simulink model "test2"  (R2024b)
settings: Solver=ode4  StartTime=0.0  StopTime=10.0  FixedStep=0.001  MaxStep=1e-3  RelTol=1e-3
settings Model: Creator=Hoan  LastModifiedBy=Hoan

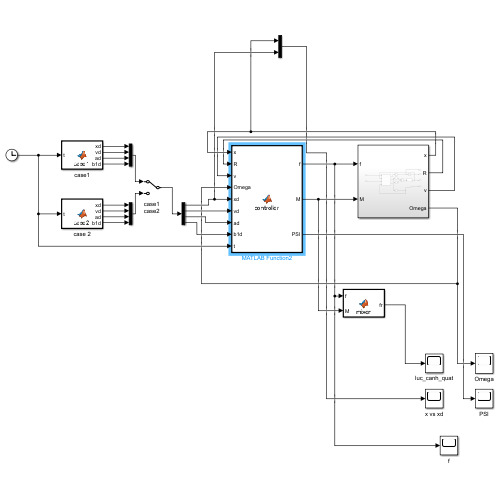
[thumbnail: Simulink's stored preview of the top-level diagram]
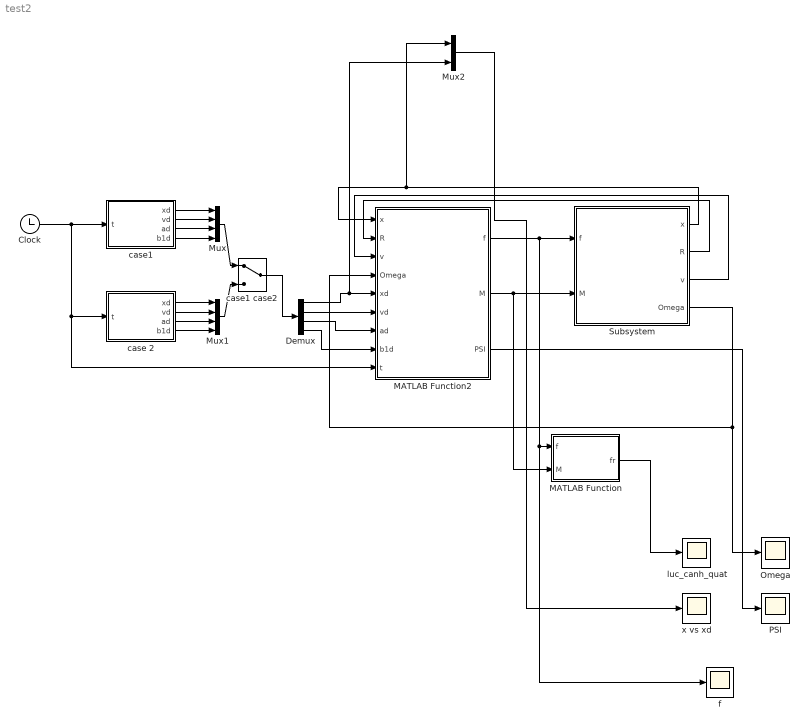
== system test2 ==
  Clock : Clock
  Demux : Demux
  MATLAB Function : MATLAB Function  TreatAsAtomicUnit=on
  MATLAB Function2 : MATLAB Function  TreatAsAtomicUnit=on
  Mux : Mux
  Mux1 : Mux
  Mux2 : Mux  Inputs=2
  Omega : Scope
  PSI : Scope
  Subsystem : Subsystem
  case 2 : MATLAB Function  TreatAsAtomicUnit=on
  case1 : MATLAB Function  TreatAsAtomicUnit=on
  "case1 case2 " : ManualSwitch
  f : Scope
  luc_canh_quat : Scope
  x vs xd : Scope
  wires:
  case1/1(xd) -> Mux/1
  case1/2(vd) -> Mux/2
  case1/3(ad) -> Mux/3
  case1/4(b1d) -> Mux/4
  case 2/1(xd) -> Mux1/1
  case 2/2(vd) -> Mux1/2
  case 2/3(ad) -> Mux1/3
  case 2/4(b1d) -> Mux1/4
  Mux/1 -> "case1 case2 "/1
  Mux1/1 -> "case1 case2 "/2
  "case1 case2 "/1 -> Demux/1
  Demux/1 -> MATLAB Function2/5(xd), Mux2/2
  Demux/3 -> MATLAB Function2/7(ad)
  Demux/2 -> MATLAB Function2/6(vd)
  Demux/4 -> MATLAB Function2/8(b1d)
  Clock/1 -> MATLAB Function2/9(t), case 2/1(t), case1/1(t)
  MATLAB Function2/1(f) -> f/1, MATLAB Function/1(f), Subsystem/1(f)
  MATLAB Function2/2(M) -> MATLAB Function/2(M), Subsystem/2(M)
  Subsystem/1(x) -> Mux2/1, MATLAB Function2/1(x)
  Subsystem/2(R) -> MATLAB Function2/2(R)
  Subsystem/4(Omega) -> MATLAB Function2/4(Omega), Omega/1
  Subsystem/3(v) -> MATLAB Function2/3(v)
  MATLAB Function/1(fr) -> luc_canh_quat/1
  MATLAB Function2/3(PSI) -> PSI/1
  Mux2/1 -> x vs xd/1

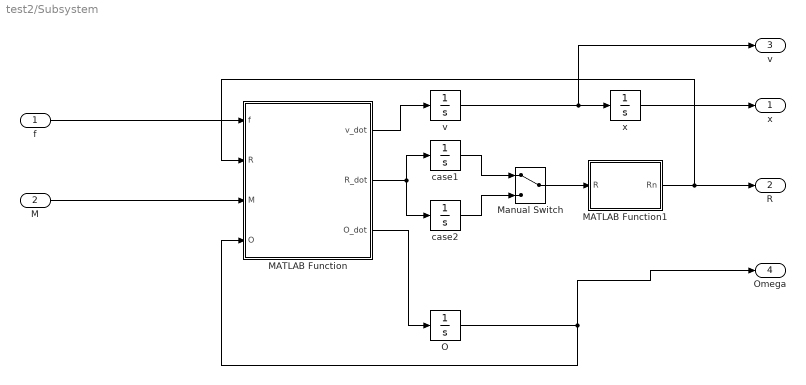
== system test2/Subsystem ==
  f : Inport
  M : Inport  Port=2
  " O" : Integrator  InitialCondition=[0;0;0]
  " v " : Integrator  InitialCondition=[0;0;0]
  " x" : Integrator  InitialCondition=[0;0;0]
  MATLAB Function : MATLAB Function  TreatAsAtomicUnit=on
  MATLAB Function1 : MATLAB Function  TreatAsAtomicUnit=on
  Manual Switch : ManualSwitch
  case1 : Integrator  InitialCondition=eye(3)
  "case2 " : Integrator  InitialCondition=[1 0 0 ; 0 -0.9995 -0.0314 ; 0 0.0314 -0.9995 ]
  x : Outport
  R : Outport  Port=2
  v : Outport  Port=3
  Omega : Outport  Port=4
  wires:
  MATLAB Function/3(O_dot) -> " O"/1
  MATLAB Function/2(R_dot) -> case1/1, "case2 "/1
  MATLAB Function/1(v_dot) -> " v "/1
  MATLAB Function1/1(Rn) -> MATLAB Function/2(R), R/1
  M/1 -> MATLAB Function/3(M)
  f/1 -> MATLAB Function/1(f)
  case1/1 -> Manual Switch/1
  "case2 "/1 -> Manual Switch/2
  Manual Switch/1 -> MATLAB Function1/1(R)
  " O"/1 -> Omega/1, MATLAB Function/4(O)
  " v "/1 -> v/1, " x"/1
  " x"/1 -> x/1

== matlab function test2/case 2 ==
  data: t input; xd output; vd output; ad output; b1d output
function [xd,vd,ad,b1d] = case2(t) %#ok<INUSD>
% Hover (Case 2)
xd  = [0;0;0];
vd  = [0;0;0];
ad  = [0;0;0];
b1d = [1;0;0];
end

== matlab function test2/case1 ==
  data: t input; xd output; vd output; ad output; b1d output
function [xd,vd,ad,b1d] = case1(t)
% Desired trajectory (Case 1)
xd = [0.4*t;0.4*sin(pi*t);-0.6*cos(pi*t)];

vd = [0.4;0.4*pi*cos(pi*t);0.6*pi*sin(pi*t)];

ad = [0;-0.4*pi*pi*sin(pi*t); 0.6*pi*pi*cos(pi*t)];

b1d = [cos(pi*t); sin(pi*t); 0];
end

== matlab function test2/MATLAB Function2 ==
  settings: updateMethod=DISCRETE
  data: x input; f output; R input; v input; Omega input; xd input; vd input; ad input; b1d input; M output; PSI output; t input
function [f, M, PSI] = controller(x, R, v, Omega, xd, vd, ad, b1d, t)
% Outputs:
%   f   : total thrust (N)
%   M   : body moment (N*m), 3x1
%   PSI : attitude configuration error function

% -------- parameters --------
m = 4.34;
g = 9.81;
J = diag([0.0820 0.0845 0.1377]);

% Gains (force-based): scale with m to keep similar closed-loop behavior
k_x = 16*m;
k_v = 5.6*m;
k_R = 8.81;
k_O = 2.54;

e3 = [0;0;1];

% -------- reshape safety --------
x     = x(:);   v     = v(:);
xd    = xd(:);  vd    = vd(:);  ad = ad(:);
Omega = Omega(:);
b1d   = b1d(:);

% -------- translational control --------
e_x = x - xd;
e_v = v - vd;

H = -k_x*e_x - k_v*e_v - m*g*e3 + m*ad;     


persistent b2d_prev
if isempty(b2d_prev)
    b2d_prev = [0;1;0];
end

% b3d
nH = norm(H);
if nH < 1e-9
    b3d = e3;
else
    b3d = -H / nH;
end

% normalize b1d
nb1 = norm(b1d);
if nb1 < 1e-9
    b1d = [1;0;0];
else
    b1d = b1d / nb1;
end

% smooth construction of b2d
Z = cross(b3d, b1d);

if norm(Z) < 1e-6
    % đừng đổi tmp đột ngột nữa, giữ hướng trước đó
    b2d = b2d_prev;
else
    b2d = Z / norm(Z);

    % giữ liên tục dấu của b2d, tránh flip 180 độ
    if dot(b2d, b2d_prev) < 0
        b2d = -b2d;
    end
end

% rebuild orthonormal basis
b1c = cross(b2d, b3d);
b1c = b1c / norm(b1c);

b2d = cross(b3d, b1c);
b2d = b2d / norm(b2d);

R_d = [b1c, b2d, b3d];

% lưu lại cho bước sau
b2d_prev = b2d;


% ensure det(Rd)=+1
[U,~,V] = svd(R_d);
R_d = U*V';
if det(R_d) < 0
    U(:,3) = -U(:,3);
    R_d = U*V';
end%

% ---------- desired angular velocity Omega_d, Omega_dot_d ----------
persistent t_prev Rd_prev Omegad_prev
if isempty(t_prev)
    t_prev = t;
    Rd_prev = R_d;
    Omegad_prev = [0;0;0];
    Omega_d = [0;0;0];
    Omega_dot_d = [0;0;0];
else
    dt = t - t_prev;
    if dt <= 1e-6
        Omega_d = Omegad_prev;
        Omega_dot_d = [0;0;0];
    else
        Rdot_d = (R_d - Rd_prev)/dt;
        W = R_d' * Rdot_d;
        W = 0.5*(W - W');      % skew
        Omega_d = vee(W);
        Omega_dot_d = (Omega_d - Omegad_prev)/dt;

        t_prev = t;
        Rd_prev = R_d;
        Omegad_prev = Omega_d;
    end
end
% -------- attitude errors --------
e_R = 0.5 * vee(R_d'*R - R'*R_d);
e_O = Omega - R'*R_d*Omega_d;

% -------- thrust and moment --------
f = -H'*(R*e3);

gyro = cross(Omega, J*Omega);
M = -k_R*e_R - k_O*e_O + gyro...
    - J*( hat(Omega)*R'*R_d*Omega_d - R'*R_d*Omega_dot_d );

% -------- PSI --------
PSI = 0.5 * trace(eye(3) - R_d'*R);

end

% ===== helpers =====
function S = hat(w)
w = w(:);
S = [   0   -w(3)  w(2);
      w(3)    0   -w(1);
     -w(2)  w(1)    0  ];
end

function w = vee(S)
w = [S(3,2); S(1,3); S(2,1)];
end

== matlab function test2/MATLAB Function ==
  data: f input; fr output; M input
function fr = mixer(f, M)
% Map total thrust & moments to rotor thrusts
% [f; Mx; My; Mz] = A * [f1; f2; f3; f4]
d = 0.315;
c = 8.004e-4;   % tau/thrust ratio (m)

A = [ 1  1  1  1;
      0 -d  0  d;
      d  0 -d  0;
      -c c -c c];

fr = A \ [f; M(:)];
end

== matlab function test2/Subsystem/MATLAB Function ==
  data: f input; v_dot output; R input; M input; O input; R_dot output; O_dot output
function [v_dot, R_dot, O_dot] = QuadDy(f, R, M, O)
% Quadrotor rigid-body dynamics (body rates)
m = 4.34;
g = 9.81;
J = diag([0.0820 0.0845 0.1377]);
e3 = [0;0;1];

O = O(:);
M = M(:);

% translation
v_dot = (m*g*e3 - f*(R*e3))/m;

% rotation kinematics
O_hat = [   0   -O(3)  O(2);
          O(3)   0   -O(1);
         -O(2)  O(1)   0  ];
R_dot = R * O_hat;

% rotational dynamics
K = cross(O, J*O);
O_dot = J \ (M - K);
end

== matlab function test2/Subsystem/MATLAB Function1 ==
  data: R input; Rn output
function Rn = NormalizeR(R)
% Project matrix to SO(3) using SVD
[U,~,V] = svd(R);
Rn = U*V';
if det(Rn) < 0
    U(:,3) = -U(:,3);
    Rn = U*V';
end
end
